simulink model "aircraft_control_model_v2"  (R2020b)
settings: Solver=ode1be  StartTime=0.0  StopTime=t  RelTol=1e-3
values from neighbouring files (symbols this model uses):
  A_ce_CG_14 = A_ce_CG_14(2:3,2:3)    [aircraft_control_model_initialisation_v2.m]
  A_ce_CG_24 = A_ce_CG_24(2:3,2:3)    [aircraft_control_model_initialisation_v2.m]
  A_ce_CG_34 = A_ce_CG_34(2:3,2:3)    [aircraft_control_model_initialisation_v2.m]
  A_sc_CG_10 = A_sc_CG_10(2:3,2:3)    [aircraft_control_model_initialisation_v2.m]
  A_sc_CG_22 = A_sc_CG_22(2:3,2:3)    [aircraft_control_model_initialisation_v2.m]
  A_sc_CG_29 = A_sc_CG_29(2:3,2:3)    [aircraft_control_model_initialisation_v2.m]
  A_sc_CG_36 = A_sc_CG_36(2:3,2:3)    [aircraft_control_model_initialisation_v2.m]
  A_sc_CG_55 = A_sc_CG_55(2:3,2:3)    [aircraft_control_model_initialisation_v2.m]
  actuator_rate = 115*pi/180    (= 2.00712863979)    [aircraft_control_model_initialisation_v2.m]
  ail_sat = 30*pi/180    (= 0.523598775598)    [aircraft_control_model_initialisation_v2.m]
  alpha0 = base_scout_aircraft_constants(16)    [aircraft_control_model_initialisation_v2.m]
  alpha0_ce = base_cessna_aircraft_constants(16)    [aircraft_control_model_initialisation_v2.m]
  alpha0tot_ce_CG_14 = consts_ce_CG_14(17)    [aircraft_control_model_initialisation_v2.m]
  alpha0tot_ce_CG_24 = consts_ce_CG_24(17)    [aircraft_control_model_initialisation_v2.m]
  alpha0tot_ce_CG_34 = consts_ce_CG_34(17)    [aircraft_control_model_initialisation_v2.m]
  alpha0tot_sc_CG_10 = consts_sc_CG_10(17)    [aircraft_control_model_initialisation_v2.m]
  alpha0tot_sc_CG_22 = consts_sc_CG_22(17)    [aircraft_control_model_initialisation_v2.m]
  alpha0tot_sc_CG_29 = consts_sc_CG_29(17)    [aircraft_control_model_initialisation_v2.m]
  alpha0tot_sc_CG_36 = consts_sc_CG_36(17)    [aircraft_control_model_initialisation_v2.m]
  alpha0tot_sc_CG_55 = consts_sc_CG_55(17)    [aircraft_control_model_initialisation_v2.m]
  alpha_ts = base_scout_aircraft_constants(19)    [aircraft_control_model_initialisation_v2.m]
  alpha_ts_ce = base_cessna_aircraft_constants(19)    [aircraft_control_model_initialisation_v2.m]
  alpha_ws = base_scout_aircraft_constants(18)    [aircraft_control_model_initialisation_v2.m]
  alpha_ws_ce = base_cessna_aircraft_constants(18)    [aircraft_control_model_initialisation_v2.m]
  AR_w = base_scout_aircraft_constants(8)    [aircraft_control_model_initialisation_v2.m]
  AR_w_ce = base_cessna_aircraft_constants(8)    [aircraft_control_model_initialisation_v2.m]
  b1 = base_scout_aircraft_constants(23)    [aircraft_control_model_initialisation_v2.m]
  b1_ce = base_cessna_aircraft_constants(23)    [aircraft_control_model_initialisation_v2.m]
  b2 = base_scout_aircraft_constants(24)    [aircraft_control_model_initialisation_v2.m]
  b2_ce = base_cessna_aircraft_constants(24)    [aircraft_control_model_initialisation_v2.m]
  b3 = base_scout_aircraft_constants(25)    [aircraft_control_model_initialisation_v2.m]
  b3_ce = base_cessna_aircraft_constants(25)    [aircraft_control_model_initialisation_v2.m]
  B_ce_CG_14 = B_ce_CG_14(2:3,1:1)    [aircraft_control_model_initialisation_v2.m]
  B_ce_CG_24 = B_ce_CG_24(2:3,1:1)    [aircraft_control_model_initialisation_v2.m]
  B_ce_CG_34 = B_ce_CG_34(2:3,1:1)    [aircraft_control_model_initialisation_v2.m]
  B_sc = B_sc(:,1)    [aircraft_control_model_initialisation_v2.m]
  B_sc_CG_10 = B_sc_CG_10(2:3,1:1)    [aircraft_control_model_initialisation_v2.m]
  B_sc_CG_22 = B_sc_CG_22(2:3,1:1)    [aircraft_control_model_initialisation_v2.m]
  B_sc_CG_29 = B_sc_CG_29(2:3,1:1)    [aircraft_control_model_initialisation_v2.m]
  B_sc_CG_36 = B_sc_CG_36(2:3,1:1)    [aircraft_control_model_initialisation_v2.m]
  B_sc_CG_55 = B_sc_CG_55(2:3,1:1)    [aircraft_control_model_initialisation_v2.m]
  beta_ce_CG_14 = consts_ce_CG_14(21)    [aircraft_control_model_initialisation_v2.m]
  beta_ce_CG_24 = consts_ce_CG_24(21)    [aircraft_control_model_initialisation_v2.m]
  beta_ce_CG_34 = consts_ce_CG_34(21)    [aircraft_control_model_initialisation_v2.m]
  beta_sc_CG_10 = consts_sc_CG_10(21)    [aircraft_control_model_initialisation_v2.m]
  beta_sc_CG_22 = consts_sc_CG_22(21)    [aircraft_control_model_initialisation_v2.m]
  beta_sc_CG_29 = consts_sc_CG_29(21)    [aircraft_control_model_initialisation_v2.m]
  beta_sc_CG_36 = consts_sc_CG_36(21)    [aircraft_control_model_initialisation_v2.m]
  beta_sc_CG_55 = consts_sc_CG_55(21)    [aircraft_control_model_initialisation_v2.m]
  c_e = base_scout_aircraft_constants(10)    [aircraft_control_model_initialisation_v2.m]
  c_e_ce = base_cessna_aircraft_constants(10)    [aircraft_control_model_initialisation_v2.m]
  Cm0 = base_scout_aircraft_constants(11)    [aircraft_control_model_initialisation_v2.m]
  control_surface_feedback = 10    [aircraft_control_model_initialisation_v2.m]
  dCL_w_dalpha = base_scout_aircraft_constants(14)    [aircraft_control_model_initialisation_v2.m]
  dCL_w_dalpha_ce = base_cessna_aircraft_constants(14)    [aircraft_control_model_initialisation_v2.m]
  dCLtot_dalpha = base_scout_aircraft_constants(15)    [aircraft_control_model_initialisation_v2.m]
  dCLtot_dalpha_ce = base_cessna_aircraft_constants(15)    [aircraft_control_model_initialisation_v2.m]
  dt = 1/100    (= 0.01)    [aircraft_control_model_initialisation_v2.m]
  elev_amplitude = 15*pi/180    (= 0.261799387799)    [aircraft_control_model_initialisation_v2.m]
  elev_cutoff = 35*pi/180    (= 0.610865238198)    [aircraft_control_model_initialisation_v2.m]
  elev_period = 1    [aircraft_control_model_initialisation_v2.m]
  elev_period_start = 5    [aircraft_control_model_initialisation_v2.m]
  elev_sat = 28*pi/180    (= 0.488692190558)    [aircraft_control_model_initialisation_v2.m]
  eta_ce_CG_14 = consts_ce_CG_14(22)    [aircraft_control_model_initialisation_v2.m]
  eta_ce_CG_24 = consts_ce_CG_24(22)    [aircraft_control_model_initialisation_v2.m]
  eta_ce_CG_34 = consts_ce_CG_34(22)    [aircraft_control_model_initialisation_v2.m]
  eta_sc_CG_10 = consts_sc_CG_10(22)    [aircraft_control_model_initialisation_v2.m]
  eta_sc_CG_22 = consts_sc_CG_22(22)    [aircraft_control_model_initialisation_v2.m]
  eta_sc_CG_29 = consts_sc_CG_29(22)    [aircraft_control_model_initialisation_v2.m]
  eta_sc_CG_36 = consts_sc_CG_36(22)    [aircraft_control_model_initialisation_v2.m]
  eta_sc_CG_55 = consts_sc_CG_55(22)    [aircraft_control_model_initialisation_v2.m]
  g = base_scout_aircraft_constants(3)    [aircraft_control_model_initialisation_v2.m]
  G = base_scout_aircraft_constants(26)    [aircraft_control_model_initialisation_v2.m]
  g_ce = base_cessna_aircraft_constants(3)    [aircraft_control_model_initialisation_v2.m]
  G_ce = base_cessna_aircraft_constants(26)    [aircraft_control_model_initialisation_v2.m]
  h0 = base_scout_aircraft_constants(13)    [aircraft_control_model_initialisation_v2.m]
  h_cg = base_scout_aircraft_constants(12)    [aircraft_control_model_initialisation_v2.m]
  K = base_scout_aircraft_constants(7)    [aircraft_control_model_initialisation_v2.m]
  l_m = base_scout_aircraft_constants(27)    [aircraft_control_model_initialisation_v2.m]
  l_m_ce = base_cessna_aircraft_constants(27)    [aircraft_control_model_initialisation_v2.m]
  m = base_scout_aircraft_constants(2)    [aircraft_control_model_initialisation_v2.m]
  m_ce = base_cessna_aircraft_constants(2)    [aircraft_control_model_initialisation_v2.m]
  modM = base_scout_aircraft_constants(30)    [aircraft_control_model_initialisation_v2.m]
  modM_ce = base_cessna_aircraft_constants(30)    [aircraft_control_model_initialisation_v2.m]
  n = base_scout_aircraft_constants(1)    [aircraft_control_model_initialisation_v2.m]    (also in xplane_data_decoder.m = data_input(6,2))
  ppgain_actuator_D = 1.076123507883140e+02    (= 107.612350788)    [aircraft_control_model_initialisation_v2.m]
  ppgain_actuator_P = 20.729870007825970    (= 20.7298700078)    [aircraft_control_model_initialisation_v2.m]
  ppgain_D = 0.637114873357555    (= 0.637114873358)    [aircraft_control_model_initialisation_v2.m]
  ppgain_P = -86.717674561182620    (= -86.7176745612)    [aircraft_control_model_initialisation_v2.m]
  r = base_scout_aircraft_constants(29)    [aircraft_control_model_initialisation_v2.m]
  r_ce = base_cessna_aircraft_constants(29)    [aircraft_control_model_initialisation_v2.m]
  rho = base_scout_aircraft_constants(4)    [aircraft_control_model_initialisation_v2.m]
  rho_ce = base_cessna_aircraft_constants(4)    [aircraft_control_model_initialisation_v2.m]
  rud_sat = 28*pi/180    (= 0.488692190558)    [aircraft_control_model_initialisation_v2.m]
  s_e = base_scout_aircraft_constants(9)    [aircraft_control_model_initialisation_v2.m]
  s_e_ce = base_cessna_aircraft_constants(9)    [aircraft_control_model_initialisation_v2.m]
  s_tp = base_scout_aircraft_constants(6)    [aircraft_control_model_initialisation_v2.m]
  s_w = base_scout_aircraft_constants(5)    [aircraft_control_model_initialisation_v2.m]
  s_w_ce = base_cessna_aircraft_constants(5)    [aircraft_control_model_initialisation_v2.m]
  tr = base_scout_aircraft_constants(28)    [aircraft_control_model_initialisation_v2.m]
  tr_ce = base_cessna_aircraft_constants(28)    [aircraft_control_model_initialisation_v2.m]
undefined symbols (not defined in the file or in its folder): A_sc
libraries: simulink x6, pid_lib x4, etargetslib x2, dspnetwork x2, aerolibanimutils x1, sldrtlib x1, cstblocks x1
(part 2 of 3)

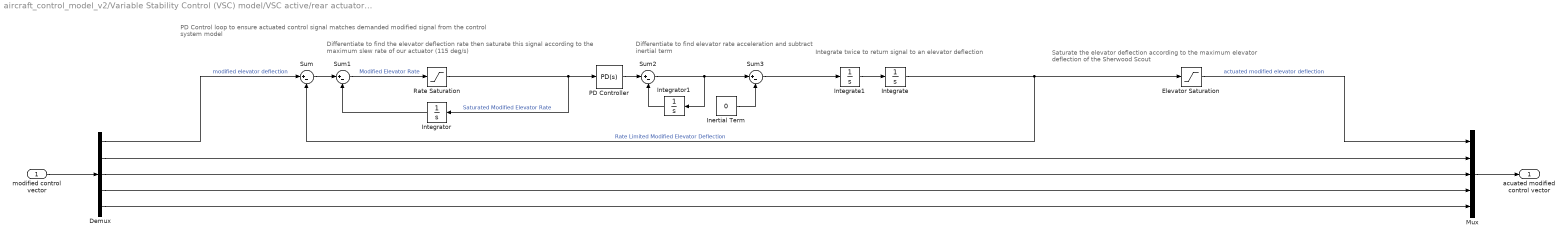
== system aircraft_control_model_v2/Variable Stability Control (VSC) model/VSC active/rear actuator model ==
  note: Differentiate to find the elevator deflection rate then saturate this signal according to the maximum slew rate of our actuator (115 deg/s)
  note: Integrate twice to return signal to an elevator deflection
  note: Saturate the elevator deflection according to the maximum elevator deflection of the Sherwood Scout
  note: PD Control loop to ensure actuated control signal matches demanded modified signal from the control system model
  note: Differentiate to find elevator rate acceleration and subtract inertial term
  modified control vector : Inport
  Demux : Demux  Outputs=5
  Elevator Saturation : Saturate  UpperLimit=elev_sat  LowerLimit=-elev_sat
  Inertial Term : Constant  Value=0
  Integrate : Integrator
  Integrate1 : Integrator
  Integrator : Integrator
  Integrator1 : Integrator
  Mux : Mux  Inputs=5
  PD Controller : pid_lib/PID Controller  Controller=PD  Form=Parallel  TimeDomain=Continuous-time  UseExternalTs=off  SampleTime=-1  IntegratorMethod=Forward Euler  FilterMethod=Forward Euler  ControllerParametersSource=internal  P=ppgain_actuator_P  I=0  D=ppgain_actuator_D  UseFilter=on  N=100  TunerSelectOption=Transfer Function Based (PID Tuner App)  InitialConditionSource=internal  InitialConditionForIntegrator=0  InitialConditionForFilter=0  DifferentiatorICPrevScaledInput=0  ExternalReset=none  TrackingMode=off  Kt=1  LimitOutput=off  SatLimitsSource=internal  UpperSaturationLimit=inf  LowerSaturationLimit=-inf  LinearizeAsGain=on  AntiWindupMode=none  Kb=1  POutMin=[]  POutMax=[]  IOutMin=[]  IOutMax=[]  DOutMin=[]  DOutMax=[]  NOutMin=[]  NOutMax=[]  SumOutMin=[]  SumOutMax=[]  SaturationOutMin=[]  SaturationOutMax=[]  PParamMin=[]  PParamMax=[]  IParamMin=[]  IParamMax=[]  DParamMin=[]  DParamMax=[]  NParamMin=[]  NParamMax=[]  KbParamMin=[]  KbParamMax=[]  KtParamMin=[]  KtParamMax=[]  KbOutMin=[]  KbOutMax=[]  KtOutMin=[]  KtOutMax=[]  IntegratorOutMin=[]  IntegratorOutMax=[]  FilterOutMin=[]  FilterOutMax=[]  SumI1OutMin=[]  SumI1OutMax=[]  SumI2OutMin=[]  SumI2OutMax=[]  SumI3OutMin=[]  SumI3OutMax=[]  SumI4OutMin=[]  SumI4OutMax=[]  SumDOutMin=[]  SumDOutMax=[]  DifferentiatorOutMin=[]  DifferentiatorOutMax=[]  FilterDiffOutCoefMin=[]  FilterDiffOutCoefMax=[]  ReciprocalOutMin=[]  ReciprocalOutMax=[]  SumDenOutMin=[]  SumDenOutMax=[]  SumNumOutMin=[]  SumNumOutMax=[]  DivideOutMin=[]  DivideOutMax=[]  UdiffTsProdOutMin=[]  UdiffTsProdOutMax=[]  NTsProdOutMin=[]  NTsProdOutMax=[]  UintegralTsProdOutMin=[]  UintegralTsProdOutMax=[]  UngainTsProdOutMin=[]  UngainTsProdOutMax=[]  IntegratorContinuousStateAttributes=''  IntegratorStateMustResolveToSignalObject=off  IntegratorRTWStateStorageClass=Auto  FilterContinuousStateAttributes=''  FilterStateMustResolveToSignalObject=off  FilterRTWStateStorageClass=Auto  ParallelPVariant=InternalParameters  IdealPVariant=Disabled  IVariant=Disabled  DVariant=InternalParameters  IntegratorVariant=Disabled  SatVariant=Disabled  AWVariant=Disabled  PCopyVariant=Disabled  TRVariant=Disabled  FdbkBlocksVariant=Forward  IdealPFdbkVariant=Disabled  SatFdbkVariant=Disabled  DerivativeFilterVariant=ContFilter  NVariant=InternalParameters  NCopyVariant=Disabled  FilterICVariant=InternalICsFilter  IntegratorICVariant=Disabled  ExternalResetVariant=Disabled  TRSumVariant=Passthrough  SumFdbkVariant=Disabled  SumVariant=Sum_PD  TsampFilterVariant=InternalTs  TsampNgainVariant=Passthrough  TsampIntegralVariant=Disabled_SignalSpec  ExternalSaturationOutDataTypeStr=Inherit: Same as second input
  Rate Saturation : Saturate  UpperLimit=actuator_rate  LowerLimit=-actuator_rate
  Sum{,1..3} (4 alike) : Sum  Inputs=|+-
  acuated modified control vector : Outport
  wires:
  Demux/1 -> Sum/1  "modified elevator deflection"
  Elevator Saturation/1 -> Mux/1  "actuated modified elevator deflection"
  Rate Saturation/1 -> Integrator/1, PD Controller/1  "Saturated Modified Elevator Rate"
  Integrate/1 -> Sum/2, Elevator Saturation/1  "Rate Limited Modified Elevator Deflection"
  Sum/1 -> Sum1/1
  Sum1/1 -> Rate Saturation/1  "Modified Elevator Rate"
  Integrator/1 -> Sum1/2
  Integrator1/1 -> Sum2/2
  PD Controller/1 -> Sum2/1
  Sum2/1 -> Sum3/1, Integrator1/1
  Inertial Term/1 -> Sum3/2
  Sum3/1 -> Integrate1/1
  Integrate1/1 -> Integrate/1
  modified control vector/1 -> Demux/1
  Demux/2 -> Mux/2
  Demux/3 -> Mux/3
  Demux/4 -> Mux/4
  Demux/5 -> Mux/5
  Mux/1 -> acuated modified control vector/1

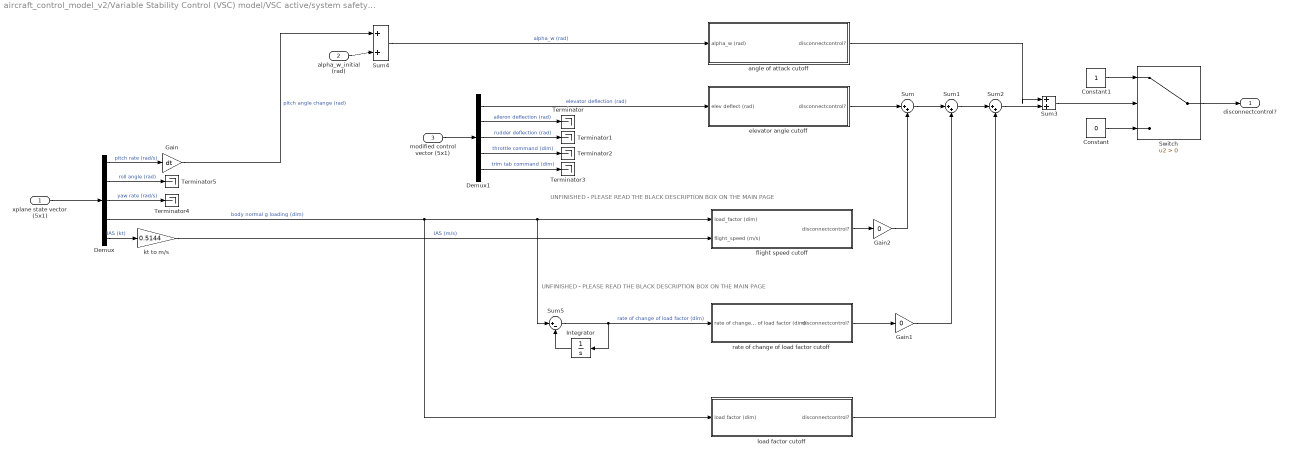
== system aircraft_control_model_v2/Variable Stability Control (VSC) model/VSC active/system safety cutoffs ==
  note: UNFINISHED - PLEASE READ THE BLACK DESCRIPTION BOX ON THE MAIN PAGE
  note: UNFINISHED - PLEASE READ THE BLACK DESCRIPTION BOX ON THE MAIN PAGE
  xplane state vector (5x1) : Inport
  alpha_w_initial (rad) : Inport  Port=2
  modified control vector (5x1) : Inport  Port=3
  Constant : Constant  Value=0
  Constant1 : Constant
  Demux : Demux  Outputs=5
  Demux1 : Demux  Outputs=5
  Gain : Gain  Gain=dt
  Gain1 : Gain  Gain=0
  Gain2 : Gain  Gain=0
  Integrator : Integrator
  Sum{,1..4} (5 alike) : Sum  Inputs=|++
  Sum5 : Sum  Inputs=|+-
  Switch : Switch  Criteria=u2 > Threshold
  Terminator{,1..5} (6 alike) : Terminator
  angle of attack cutoff : Subsystem
  elevator angle cutoff : Subsystem
  flight speed cutoff : Subsystem
  kt to m/s : Gain  Gain=0.5144
  load factor cutoff : Subsystem
  rate of change of load factor cutoff : Subsystem
  disconnectcontrol? : Outport
  wires:
  elevator angle cutoff/1(disconnectcontrol?) -> Sum/1
  Constant/1 -> Switch/3
  Constant1/1 -> Switch/1
  Switch/1 -> disconnectcontrol?/1
  Sum/1 -> Sum1/1
  Sum1/1 -> Sum2/1
  Sum2/1 -> Sum3/2
  rate of change of load factor cutoff/1(disconnectcontrol?) -> Gain1/1
  load factor cutoff/1(disconnectcontrol?) -> Sum2/2
  angle of attack cutoff/1(disconnectcontrol?) -> Sum3/1
  Sum4/1 -> angle of attack cutoff/1(alpha_w (rad))  "alpha_w (rad)"
  xplane state vector (5x1)/1 -> Demux/1
  Demux/1 -> Gain/1  "pitch rate (rad/s)"
  Demux/4 -> load factor cutoff/1(load factor (dim)), Sum5/1, flight speed cutoff/1(load_factor (dim))  "body normal g loading (dim)"
  Demux/2 -> Terminator5/1  "roll angle (rad)"
  Demux/3 -> Terminator4/1  "yaw rate (rad/s)"
  Demux/5 -> kt to m/s/1  "IAS (kt)"
  kt to m/s/1 -> flight speed cutoff/2(flight_speed (m/s))  "IAS (m/s)"
  modified control vector (5x1)/1 -> Demux1/1
  Demux1/1 -> elevator angle cutoff/1(elev deflect (rad))  "elevator deflection (rad)"
  Demux1/2 -> Terminator/1  "aileron deflection (rad)"
  Demux1/3 -> Terminator1/1  "rudder deflection (rad)"
  Demux1/4 -> Terminator2/1  "throttle command (dim)"
  Demux1/5 -> Terminator3/1  "trim tab command (dim)"
  alpha_w_initial (rad)/1 -> Sum4/2
  Gain/1 -> Sum4/1  "pitch angle change (rad)"
  Integrator/1 -> Sum5/2
  Sum5/1 -> Integrator/1, rate of change of load factor cutoff/1(rate of change of load factor (dim))  "rate of change of load factor (dim)"
  flight speed cutoff/1(disconnectcontrol?) -> Gain2/1
  Sum3/1 -> Switch/2
  Gain1/1 -> Sum1/2
  Gain2/1 -> Sum/2

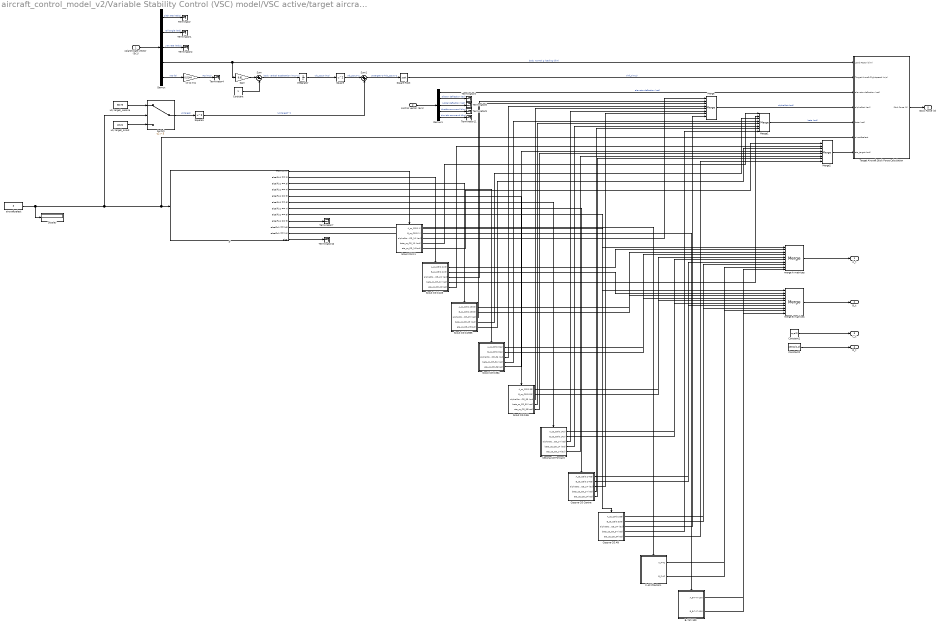
== system aircraft_control_model_v2/Variable Stability Control (VSC) model/VSC active/target aircraft state space selection ==
  xplane state vector (5x1) : Inport
  control vector (5x1) : Inport  Port=2
  B-747-100 : Subsystem  TreatAsAtomicUnit=on
  Cessna CG Aft : Subsystem  TreatAsAtomicUnit=on
  Cessna CG Centre : Subsystem  TreatAsAtomicUnit=on
  Cessna CG Forward : Subsystem  TreatAsAtomicUnit=on
  Constant : Constant
  Constant1 : Constant  Value=eye(2)
  Constant2 : Constant  Value=zeros(1,2)
  Demux : Demux  Outputs=5
  Demux1 : Demux  Outputs=5
  Display : Display
  F-4C Phantom : Subsystem  TreatAsAtomicUnit=on
  Gain : Gain  Gain=9.81
  If : If  IfExpression=u1 == 1  ElseIfExpressions=u1 == 2, u1 == 3, u1 == 4, u1 == 5, u1 == 6, u1 == 7, u1 == 8, u1 == 9, u1 == 10, u1 == 11
  Integrator : Integrator
  Merge : Merge  Inputs=8
  Merge1 : Merge  Inputs=8
  Merge2 : Merge  Inputs=8
  Scout CG 0.1 : Subsystem  TreatAsAtomicUnit=on
  Scout CG 0.223 : Subsystem  TreatAsAtomicUnit=on
  Scout CG 0.2935 : Subsystem  TreatAsAtomicUnit=on
  Scout CG 0.364 : Subsystem  TreatAsAtomicUnit=on
  Scout CG 0.55 : Subsystem  TreatAsAtomicUnit=on
  Square : Math  Operator=square  SaturateOnIntegerOverflow=on
  Square Root : Sqrt  SaturateOnIntegerOverflow=on
  Square1 : Math  Operator=square  SaturateOnIntegerOverflow=on
  Sum : Sum  Inputs=|+-
  Sum1 : Sum  Inputs=|++
  Switch : Switch  Criteria=u2 > Threshold  Threshold=5
  Target Aircraft Stick Force Calculation : Subsystem
  Terminator{,1..4,7..11} (10 alike) : Terminator
  aircraftselect : Constant  Value=3
  kt to m/s : Gain  Gain=0.5144
  merge A matrices : Merge  Inputs=10
  merge B matrices : Merge  Inputs=10
  "u0, target_cessna" : Constant  Value=66.75
  "u0, target_scout" : Constant  Value=43.21
  A_t : Outport
  B_t : Outport  Port=2
  C_t : Outport  Port=3
  D_t : Outport  Port=4
  Stick Force (N) : Outport  Port=5
  wires:
  If/1 -> Scout CG 0.1/Action
  If/2 -> Scout CG 0.223/Action
  If/3 -> Scout CG 0.2935/Action
  If/4 -> Scout CG 0.364/Action
  If/5 -> Scout CG 0.55/Action
  If/6 -> Cessna CG Forward/Action
  If/7 -> Cessna CG Centre/Action
  If/8 -> Cessna CG Aft/Action
  If/9 -> Terminator7/1
  If/10 -> F-4C Phantom/Action
  If/11 -> B-747-100/Action
  If/12 -> Terminator10/1
  Scout CG 0.1/1(A_sc_CG(0.1)) -> merge A matrices/1
  Scout CG 0.223/1(A_sc_CG(0.223)) -> merge A matrices/2
  merge A matrices/1 -> A_t/1
  merge B matrices/1 -> B_t/1
  Scout CG 0.1/2(B_sc_CG(0.1)) -> merge B matrices/1
  Scout CG 0.223/2(B_sc_CG(0.223)) -> merge B matrices/2
  Constant1/1 -> C_t/1
  Constant2/1 -> D_t/1
  aircraftselect/1 -> Display/1, If/1, Target Aircraft Stick Force Calculation/6(aircraftselect), Switch/2
  Scout CG 0.2935/1(A_sc_CG(0.2935)) -> merge A matrices/3
  Scout CG 0.2935/2(B_sc_CG(0.2935)) -> merge B matrices/3
  Scout CG 0.364/1(A_sc_CG(0.364)) -> merge A matrices/4
  Scout CG 0.364/2(B_sc_CG(0.364)) -> merge B matrices/4
  Scout CG 0.55/1(A_sc_CG(0.55)) -> merge A matrices/5
  Scout CG 0.55/2(B_sc_CG(0.55)) -> merge B matrices/5
  xplane state vector (5x1)/1 -> Demux/1
  Demux/5 -> kt to m/s/1  "IAS (kt)"
  Demux/1 -> Terminator/1  "pitch rate (rad/s)"
  Demux/2 -> Terminator1/1  "roll angle (rad)"
  Demux/3 -> Terminator2/1  "yaw rate (rad/s)"
  Demux/4 -> Target Aircraft Stick Force Calculation/1(Load Factor (dim)), Gain/1  "body normal g loading (dim)"
  kt to m/s/1 -> Terminator4/1  "IAS (m/s)"
  control vector (5x1)/1 -> Demux1/1
  Demux1/1 -> Target Aircraft Stick Force Calculation/3(elevator deflection (rad))  "elevator deflection (rad)"
  Demux1/2 -> Terminator3/1  "aileron deflection (rad)"
  Demux1/3 -> Terminator8/1  "rudder deflection (rad)"
  Demux1/4 -> Terminator9/1  "throttle command (dim)"
  Demux1/5 -> Terminator11/1  "trim tab command (dim)"
  Merge/1 -> Target Aircraft Stick Force Calculation/4(alpha0tot (rad))  "alpha0tot (rad)"
  Merge1/1 -> Target Aircraft Stick Force Calculation/5(beta (rad))  "beta (rad)"
  Scout CG 0.223/3(alpha0tot_sc_CG_22 (rad)) -> Merge/2
  Scout CG 0.1/3(alpha0tot_sc_CG_10 (rad)) -> Merge/1
  Scout CG 0.2935/3(alpha0tot_sc_CG_29 (rad)) -> Merge/3
  Scout CG 0.364/3(alpha0tot_sc_CG_36 (rad)) -> Merge/4
  Scout CG 0.55/3(alpha0tot_sc_CG_55 (rad)) -> Merge/5
  Scout CG 0.1/4(beta_sc_CG_10 (rad)) -> Merge1/1
  Scout CG 0.223/4(beta_sc_CG_22 (rad)) -> Merge1/2
  Scout CG 0.2935/4(beta_sc_CG_29 (rad)) -> Merge1/3
  Scout CG 0.364/4(beta_sc_CG_36 (rad)) -> Merge1/4
  Scout CG 0.55/4(beta_sc_CG_55 (rad)) -> Merge1/5
  Target Aircraft Stick Force Calculation/1(Stick Force (N)) -> Stick Force (N)/1
  Cessna CG Forward/1(A_ce_CG(0.143)) -> merge A matrices/6
  Cessna CG Centre/1(A_ce_CG(0.2405)) -> merge A matrices/7
  Cessna CG Aft/1(A_ce_CG(0.338)) -> merge A matrices/8
  F-4C Phantom/1(A_F-4C) -> merge A matrices/9
  B-747-100/1(A_B-747-100) -> merge A matrices/10
  Cessna CG Forward/2(B_ce_CG(0.143)) -> merge B matrices/6
  Cessna CG Centre/2(B_ce_CG(0.2405)) -> merge B matrices/7
  Cessna CG Aft/2(B_ce_CG(0.338)) -> merge B matrices/8
  F-4C Phantom/2(B_F-4C) -> merge B matrices/9
  B-747-100/2(B_B-747-100) -> merge B matrices/10
  Cessna CG Forward/3(alpha0tot_ce_CG_14 (rad)) -> Merge/6
  Cessna CG Centre/3(alpha0tot_ce_CG_24 (rad)) -> Merge/7
  Cessna CG Aft/3(alpha0tot_ce_CG_34 (rad)) -> Merge/8
  Cessna CG Forward/4(beta_ce_CG_14 (rad)) -> Merge1/6
  Cessna CG Centre/4(beta_ce_CG_24 (rad)) -> Merge1/7
  Cessna CG Aft/4(beta_ce_CG_34 (rad)) -> Merge1/8
  Merge2/1 -> Target Aircraft Stick Force Calculation/7(eta_target (rad))
  Scout CG 0.1/5(eta_sc_CG_10(rad)) -> Merge2/1
  Scout CG 0.223/5(eta_sc_CG_22(rad)) -> Merge2/2
  Scout CG 0.2935/5(eta_sc_CG_29(rad)) -> Merge2/3
  Scout CG 0.364/5(eta_sc_CG_36(rad)) -> Merge2/4
  Scout CG 0.55/5(eta_sc_CG_55(rad)) -> Merge2/5
  Cessna CG Forward/5(eta_ce_CG_14(rad)) -> Merge2/6
  Cessna CG Centre/5(eta_ce_CG_24(rad)) -> Merge2/7
  Cessna CG Aft/5(eta_ce_CG_34(rad)) -> Merge2/8
  "u0, target_cessna"/1 -> Switch/1
  "u0, target_scout"/1 -> Switch/3
  Switch/1 -> Square1/1  "u0,target"
  Gain/1 -> Sum/1
  Constant/1 -> Sum/2
  Sum/1 -> Integrator/1  "body vertical acceleration (m/s^2)"
  Integrator/1 -> Square/1  "wb_scout (m/s)"
  Square/1 -> Sum1/1  "wb_scout^2"
  Square1/1 -> Sum1/2  "(u0,target)^2"
  Sum1/1 -> Square Root/1  "u0,target^2+wb_scout^2"
  Square Root/1 -> Target Aircraft Stick Force Calculation/2(Target Aircraft Flightspeed (m/s))  "Vinf_t (m/s)"

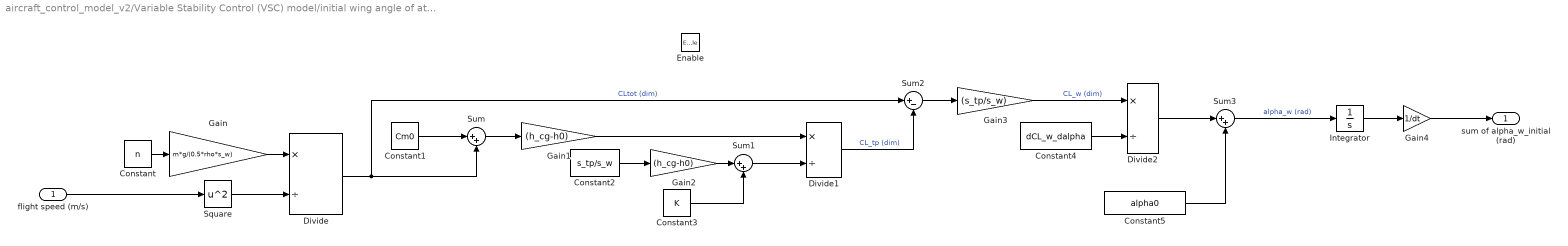
== system aircraft_control_model_v2/Variable Stability Control (VSC) model/initial wing angle of attack (rad) estimation/Enabled Subsystem ==
  flight speed (m/s) : Inport
  Enable : EnablePort
  Constant : Constant  Value=n
  Constant1 : Constant  Value=Cm0
  Constant2 : Constant  Value=s_tp/s_w
  Constant3 : Constant  Value=K
  Constant4 : Constant  Value=dCL_w_dalpha
  Constant5 : Constant  Value=alpha0
  Divide : Product  Inputs=*/
  Divide1 : Product  Inputs=*/
  Divide2 : Product  Inputs=*/
  Gain : Gain  Gain=m*g/(0.5*rho*s_w)
  Gain1 : Gain  Gain=(h_cg-h0)
  Gain2 : Gain  Gain=(h_cg-h0)
  Gain3 : Gain  Gain=(s_tp/s_w)
  Gain4 : Gain  Gain=1/dt
  Integrator : Integrator
  Square : Math  Operator=square  SaturateOnIntegerOverflow=on
  Sum : Sum  Inputs=|++
  Sum1 : Sum  Inputs=|++
  Sum2 : Sum  Inputs=|+-
  Sum3 : Sum  Inputs=|++
  sum of alpha_w_initial (rad) : Outport
  wires:
  Gain1/1 -> Divide1/1
  Gain/1 -> Divide/1
  Gain2/1 -> Sum1/1
  Divide/1 -> Sum2/1, Sum/2  "CLtot (dim)"
  Constant/1 -> Gain/1
  Sum/1 -> Gain1/1
  Constant4/1 -> Divide2/2
  Divide2/1 -> Sum3/1
  Constant3/1 -> Sum1/2
  Sum1/1 -> Divide1/2
  Sum2/1 -> Gain3/1
  Constant1/1 -> Sum/1
  Square/1 -> Divide/2
  Constant2/1 -> Gain2/1
  Gain3/1 -> Divide2/1  "CL_w (dim)"
  Constant5/1 -> Sum3/2
  Sum3/1 -> Integrator/1  "alpha_w (rad)"
  flight speed (m/s)/1 -> Square/1
  Divide1/1 -> Sum2/2  "CL_tp (dim)"
  Integrator/1 -> Gain4/1
  Gain4/1 -> sum of alpha_w_initial (rad)/1

== system aircraft_control_model_v2/Control Inputs/pilot joystick input/control surface commands to control surface deflections/aileron command to aileron deflection ==
  aileron command (dim) : Inport
  Gain2 : Gain  Gain=control_surface_feedback
  Gain3 : Gain  Gain=control_surface_feedback*(ail_sat)
  Integrator4 : Integrator
  Sum1 : Sum  Inputs=|+-
  aileron deflection (rad) : Outport
  wires:
  Gain2/1 -> Sum1/2
  Sum1/1 -> Integrator4/1
  Gain3/1 -> aileron deflection (rad)/1  "aileron deflection (rad)"
  Integrator4/1 -> Gain3/1, Gain2/1
  aileron command (dim)/1 -> Sum1/1

== system aircraft_control_model_v2/Control Inputs/pilot joystick input/control surface commands to control surface deflections/elevator command to elevator deflection ==
  elevator command (dim) : Inport
  Gain : Gain  Gain=control_surface_feedback
  Gain1 : Gain  Gain=control_surface_feedback*(elev_sat)
  Gain2 : Gain  Gain=-1
  Integrator1 : Integrator
  Sum : Sum  Inputs=|+-
  elevator deflection (rad) : Outport
  wires:
  Integrator1/1 -> Gain/1, Gain1/1
  Gain1/1 -> elevator deflection (rad)/1  "elevator deflection (rad)"
  Sum/1 -> Integrator1/1
  Gain/1 -> Sum/2
  elevator command (dim)/1 -> Gain2/1
  Gain2/1 -> Sum/1

== system aircraft_control_model_v2/Control Inputs/pilot joystick input/control surface commands to control surface deflections/rudder command to rudder deflection ==
  rudder command (dim) : Inport
  Gain4 : Gain  Gain=control_surface_feedback
  Gain5 : Gain  Gain=control_surface_feedback*(rud_sat)
  Integrator3 : Integrator
  Sum2 : Sum  Inputs=|+-
  rudder deflection (rad) : Outport
  wires:
  Integrator3/1 -> Gain5/1, Gain4/1
  Gain5/1 -> rudder deflection (rad)/1  "rudder deflection (rad)"
  Sum2/1 -> Integrator3/1
  Gain4/1 -> Sum2/2
  rudder command (dim)/1 -> Sum2/1

== system aircraft_control_model_v2/Variable Stability Control (VSC) model/VSC active/system safety cutoffs/angle of attack cutoff ==
  alpha_w (rad) : Inport
  +ve wing angle of attack limit (rad) : simulink/Logic and Bit Operations/Compare To Constant  relop=>  const=10*pi/180  OutDataTypeStr=boolean
  -ve wing angle of attack limit (rad) : simulink/Logic and Bit Operations/Compare To Constant  relop=<  const=-7*pi/180  OutDataTypeStr=boolean
  Constant : Constant  Value=0
  Constant1 : Constant
  Logical Operator : Logic  Operator=OR  AllPortsSameDT=off  OutDataTypeStr=boolean
  Logical Operator1 : Logic  Operator=OR  AllPortsSameDT=off  OutDataTypeStr=boolean
  Memory : Memory
  Memory1 : Memory
  Sum : Sum  Inputs=|++
  Switch : Switch  Criteria=u2 > Threshold
  disconnectcontrol? : Outport
  wires:
  Constant/1 -> Switch/3
  Constant1/1 -> Switch/1
  Logical Operator/1 -> Sum/1, Memory/1
  Memory/1 -> Logical Operator/1
  Sum/1 -> Switch/2
  Logical Operator1/1 -> Sum/2, Memory1/1
  +ve wing angle of attack limit (rad)/1 -> Logical Operator/2
  -ve wing angle of attack limit (rad)/1 -> Logical Operator1/2
  alpha_w (rad)/1 -> -ve wing angle of attack limit (rad)/1, +ve wing angle of attack limit (rad)/1
  Memory1/1 -> Logical Operator1/1
  Switch/1 -> disconnectcontrol?/1

== system aircraft_control_model_v2/Variable Stability Control (VSC) model/VSC active/system safety cutoffs/elevator angle cutoff ==
  elev deflect (rad) : Inport
  Abs : Abs
  Compare To Constant : simulink/Logic and Bit Operations/Compare To Constant  relop=>  const=elev_cutoff  OutDataTypeStr=boolean
  Logical Operator : Logic  Operator=OR  AllPortsSameDT=off  OutDataTypeStr=boolean
  Memory : Memory
  disconnectcontrol? : Outport
  wires:
  Memory/1 -> Logical Operator/1
  elev deflect (rad)/1 -> Abs/1
  Abs/1 -> Compare To Constant/1
  Compare To Constant/1 -> Logical Operator/2
  Logical Operator/1 -> disconnectcontrol?/1, Memory/1

== system aircraft_control_model_v2/Variable Stability Control (VSC) model/VSC active/system safety cutoffs/flight speed cutoff ==
  load_factor (dim) : Inport
  flight_speed (m/s) : Inport  Port=2
  Logical Operator1 : Logic  Operator=OR  AllPortsSameDT=off  OutDataTypeStr=boolean
  MATLAB Function : MATLAB Function  TreatAsAtomicUnit=on
  Memory1 : Memory
  Relational Operator : RelationalOperator  Operator=<  OutDataTypeStr=boolean  RndMeth=Simplest
  disconnectcontrol? : Outport
  wires:
  load_factor (dim)/1 -> MATLAB Function/1(n)  "Load Factor (dim)"
  flight_speed (m/s)/1 -> Relational Operator/1  "flight_speed (m/s)"
  Relational Operator/1 -> Logical Operator1/2
  Memory1/1 -> Logical Operator1/1
  Logical Operator1/1 -> disconnectcontrol?/1, Memory1/1
  MATLAB Function/1(Va) -> Relational Operator/2

== system aircraft_control_model_v2/Variable Stability Control (VSC) model/VSC active/system safety cutoffs/load factor cutoff ==
  load factor (dim) : Inport
  Compare To Constant : simulink/Logic and Bit Operations/Compare To Constant  relop=>  const=3.5  OutDataTypeStr=boolean
  Compare To Constant1 : simulink/Logic and Bit Operations/Compare To Constant  relop=<  const=-1.2  OutDataTypeStr=boolean
  Constant : Constant  Value=0
  Constant1 : Constant
  Logical Operator : Logic  Operator=OR  AllPortsSameDT=off  OutDataTypeStr=boolean
  Logical Operator1 : Logic  Operator=OR  AllPortsSameDT=off  OutDataTypeStr=boolean
  Memory : Memory
  Memory1 : Memory
  Sum : Sum  Inputs=|++
  Switch : Switch  Criteria=u2 > Threshold
  disconnectcontrol? : Outport
  wires:
  load factor (dim)/1 -> Compare To Constant1/1, Compare To Constant/1
  Compare To Constant/1 -> Logical Operator/2
  Memory/1 -> Logical Operator/1
  Logical Operator/1 -> Sum/1, Memory/1
  Compare To Constant1/1 -> Logical Operator1/2
  Memory1/1 -> Logical Operator1/1
  Logical Operator1/1 -> Sum/2, Memory1/1
  Sum/1 -> Switch/2
  Constant1/1 -> Switch/1
  Constant/1 -> Switch/3
  Switch/1 -> disconnectcontrol?/1

== system aircraft_control_model_v2/Variable Stability Control (VSC) model/VSC active/system safety cutoffs/rate of change of load factor cutoff ==
  rate of change of load factor (dim) : Inport
  Abs : Abs
  Compare To Constant : simulink/Logic and Bit Operations/Compare To Constant  relop=>  const=7.8  OutDataTypeStr=boolean
  Logical Operator : Logic  Operator=OR  AllPortsSameDT=off  OutDataTypeStr=boolean
  Memory : Memory
  disconnectcontrol? : Outport
  wires:
  Logical Operator/1 -> disconnectcontrol?/1, Memory/1
  Abs/1 -> Compare To Constant/1
  Compare To Constant/1 -> Logical Operator/2
  Memory/1 -> Logical Operator/1
  rate of change of load factor (dim)/1 -> Abs/1

== system aircraft_control_model_v2/Variable Stability Control (VSC) model/VSC active/target aircraft state space selection/B-747-100 ==
  Action Port : ActionPort  ActionPortLabel=elseif( u1 == 11)
  Constant : Constant  Value=|
      | [-0.508647705600000	65.0870077697200
      | -0.00557351174471139	-0.415074491893133]
  Constant1 : Constant  Value=|
      | [-1.97021509716000
      | -0.377425932894150]
  A_B-747-100 : Outport
  B_B-747-100 : Outport  Port=2
  wires:
  Constant/1 -> A_B-747-100/1
  Constant1/1 -> B_B-747-100/1

== system aircraft_control_model_v2/Variable Stability Control (VSC) model/VSC active/target aircraft state space selection/Cessna CG Aft ==
  Action Port : ActionPort  ActionPortLabel=elseif( u1 == 8)
  Constant : Constant  Value=A_ce_CG_34
  Constant1 : Constant  Value=B_ce_CG_34
  Constant2 : Constant  Value=alpha0tot_ce_CG_34
  Constant3 : Constant  Value=beta_ce_CG_34
  Constant4 : Constant  Value=eta_ce_CG_34
  A_ce_CG(0.338) : Outport
  B_ce_CG(0.338) : Outport  Port=2
  alpha0tot_ce_CG_34 (rad) : Outport  Port=3
  beta_ce_CG_34 (rad) : Outport  Port=4
  eta_ce_CG_34(rad) : Outport  Port=5
  wires:
  Constant/1 -> A_ce_CG(0.338)/1
  Constant1/1 -> B_ce_CG(0.338)/1
  Constant2/1 -> alpha0tot_ce_CG_34 (rad)/1
  Constant3/1 -> beta_ce_CG_34 (rad)/1
  Constant4/1 -> eta_ce_CG_34(rad)/1

== system aircraft_control_model_v2/Variable Stability Control (VSC) model/VSC active/target aircraft state space selection/Cessna CG Centre ==
  Action Port : ActionPort  ActionPortLabel=elseif( u1 == 7)
  Constant : Constant  Value=A_ce_CG_24
  Constant1 : Constant  Value=B_ce_CG_24
  Constant2 : Constant  Value=alpha0tot_ce_CG_24
  Constant3 : Constant  Value=beta_ce_CG_24
  Constant4 : Constant  Value=eta_ce_CG_24
  A_ce_CG(0.2405) : Outport
  B_ce_CG(0.2405) : Outport  Port=2
  alpha0tot_ce_CG_24 (rad) : Outport  Port=3
  beta_ce_CG_24 (rad) : Outport  Port=4
  eta_ce_CG_24(rad) : Outport  Port=5
  wires:
  Constant/1 -> A_ce_CG(0.2405)/1
  Constant1/1 -> B_ce_CG(0.2405)/1
  Constant2/1 -> alpha0tot_ce_CG_24 (rad)/1
  Constant3/1 -> beta_ce_CG_24 (rad)/1
  Constant4/1 -> eta_ce_CG_24(rad)/1

== system aircraft_control_model_v2/Variable Stability Control (VSC) model/VSC active/target aircraft state space selection/Cessna CG Forward ==
  Action Port : ActionPort  ActionPortLabel=elseif( u1 == 6)
  Constant : Constant  Value=A_ce_CG_14
  Constant1 : Constant  Value=B_ce_CG_14
  Constant2 : Constant  Value=alpha0tot_ce_CG_14
  Constant3 : Constant  Value=beta_ce_CG_14
  Constant4 : Constant  Value=eta_ce_CG_14
  A_ce_CG(0.143) : Outport
  B_ce_CG(0.143) : Outport  Port=2
  alpha0tot_ce_CG_14 (rad) : Outport  Port=3
  beta_ce_CG_14 (rad) : Outport  Port=4
  eta_ce_CG_14(rad) : Outport  Port=5
  wires:
  Constant/1 -> A_ce_CG(0.143)/1
  Constant1/1 -> B_ce_CG(0.143)/1
  Constant2/1 -> alpha0tot_ce_CG_14 (rad)/1
  Constant3/1 -> beta_ce_CG_14 (rad)/1
  Constant4/1 -> eta_ce_CG_14(rad)/1

== system aircraft_control_model_v2/Variable Stability Control (VSC) model/VSC active/target aircraft state space selection/F-4C Phantom ==
  Action Port : ActionPort  ActionPortLabel=elseif( u1 == 10)
  Constant : Constant  Value=|
      | [-0.295319442940517	177.255749314106
      | -0.0104482212700093	-0.448358567032906]
  Constant1 : Constant  Value=|
      | [-6.29389106785740
      | -4.88848338612147]
  A_F-4C : Outport
  B_F-4C : Outport  Port=2
  wires:
  Constant/1 -> A_F-4C/1
  Constant1/1 -> B_F-4C/1

== system aircraft_control_model_v2/Variable Stability Control (VSC) model/VSC active/target aircraft state space selection/Scout CG 0.1 ==
  Action Port : ActionPort  ActionPortLabel=if(u1 == 1)
  Constant : Constant  Value=A_sc_CG_10
  Constant1 : Constant  Value=B_sc_CG_10
  Constant2 : Constant  Value=alpha0tot_sc_CG_10
  Constant3 : Constant  Value=beta_sc_CG_10
  Constant4 : Constant  Value=eta_sc_CG_10
  A_sc_CG(0.1) : Outport
  B_sc_CG(0.1) : Outport  Port=2
  alpha0tot_sc_CG_10 (rad) : Outport  Port=3
  beta_sc_CG_10 (rad) : Outport  Port=4
  eta_sc_CG_10(rad) : Outport  Port=5
  wires:
  Constant/1 -> A_sc_CG(0.1)/1
  Constant1/1 -> B_sc_CG(0.1)/1
  Constant2/1 -> alpha0tot_sc_CG_10 (rad)/1
  Constant3/1 -> beta_sc_CG_10 (rad)/1
  Constant4/1 -> eta_sc_CG_10(rad)/1

== system aircraft_control_model_v2/Variable Stability Control (VSC) model/VSC active/target aircraft state space selection/Scout CG 0.223 ==
  Action Port : ActionPort  ActionPortLabel=elseif(u1 == 2)
  Constant : Constant  Value=A_sc_CG_22
  Constant1 : Constant  Value=B_sc_CG_22
  Constant2 : Constant  Value=alpha0tot_sc_CG_22
  Constant3 : Constant  Value=beta_sc_CG_22
  Constant4 : Constant  Value=eta_sc_CG_22
  A_sc_CG(0.223) : Outport
  B_sc_CG(0.223) : Outport  Port=2
  alpha0tot_sc_CG_22 (rad) : Outport  Port=3
  beta_sc_CG_22 (rad) : Outport  Port=4
  eta_sc_CG_22(rad) : Outport  Port=5
  wires:
  Constant/1 -> A_sc_CG(0.223)/1
  Constant1/1 -> B_sc_CG(0.223)/1
  Constant2/1 -> alpha0tot_sc_CG_22 (rad)/1
  Constant3/1 -> beta_sc_CG_22 (rad)/1
  Constant4/1 -> eta_sc_CG_22(rad)/1

== system aircraft_control_model_v2/Variable Stability Control (VSC) model/VSC active/target aircraft state space selection/Scout CG 0.2935 ==
  Action Port : ActionPort  ActionPortLabel=elseif( u1 == 3)
  Constant : Constant  Value=A_sc_CG_29
  Constant1 : Constant  Value=B_sc_CG_29
  Constant2 : Constant  Value=alpha0tot_sc_CG_29
  Constant3 : Constant  Value=beta_sc_CG_29
  Constant4 : Constant  Value=eta_sc_CG_29
  A_sc_CG(0.2935) : Outport
  B_sc_CG(0.2935) : Outport  Port=2
  alpha0tot_sc_CG_29 (rad) : Outport  Port=3
  beta_sc_CG_29 (rad) : Outport  Port=4
  eta_sc_CG_29(rad) : Outport  Port=5
  wires:
  Constant/1 -> A_sc_CG(0.2935)/1
  Constant1/1 -> B_sc_CG(0.2935)/1
  Constant2/1 -> alpha0tot_sc_CG_29 (rad)/1
  Constant3/1 -> beta_sc_CG_29 (rad)/1
  Constant4/1 -> eta_sc_CG_29(rad)/1

== system aircraft_control_model_v2/Variable Stability Control (VSC) model/VSC active/target aircraft state space selection/Scout CG 0.364 ==
  Action Port : ActionPort  ActionPortLabel=elseif( u1 == 4)
  Constant : Constant  Value=A_sc_CG_36
  Constant1 : Constant  Value=B_sc_CG_36
  Constant2 : Constant  Value=alpha0tot_sc_CG_36
  Constant3 : Constant  Value=beta_sc_CG_36
  Constant4 : Constant  Value=eta_sc_CG_36
  A_sc_CG(0.364) : Outport
  B_sc_CG(0.364) : Outport  Port=2
  alpha0tot_sc_CG_36 (rad) : Outport  Port=3
  beta_sc_CG_36 (rad) : Outport  Port=4
  eta_sc_CG_36(rad) : Outport  Port=5
  wires:
  Constant/1 -> A_sc_CG(0.364)/1
  Constant1/1 -> B_sc_CG(0.364)/1
  Constant2/1 -> alpha0tot_sc_CG_36 (rad)/1
  Constant3/1 -> beta_sc_CG_36 (rad)/1
  Constant4/1 -> eta_sc_CG_36(rad)/1

== system aircraft_control_model_v2/Variable Stability Control (VSC) model/VSC active/target aircraft state space selection/Scout CG 0.55 ==
  Action Port : ActionPort  ActionPortLabel=elseif( u1 == 5)
  Constant : Constant  Value=A_sc_CG_55
  Constant1 : Constant  Value=B_sc_CG_55
  Constant2 : Constant  Value=alpha0tot_sc_CG_55
  Constant3 : Constant  Value=beta_sc_CG_55
  Constant4 : Constant  Value=eta_sc_CG_55
  A_sc_CG(0.55) : Outport
  B_sc_CG(0.55) : Outport  Port=2
  alpha0tot_sc_CG_55 (rad) : Outport  Port=3
  beta_sc_CG_55 (rad) : Outport  Port=4
  eta_sc_CG_55(rad) : Outport  Port=5
  wires:
  Constant/1 -> A_sc_CG(0.55)/1
  Constant1/1 -> B_sc_CG(0.55)/1
  Constant2/1 -> alpha0tot_sc_CG_55 (rad)/1
  Constant3/1 -> beta_sc_CG_55 (rad)/1
  Constant4/1 -> eta_sc_CG_55(rad)/1

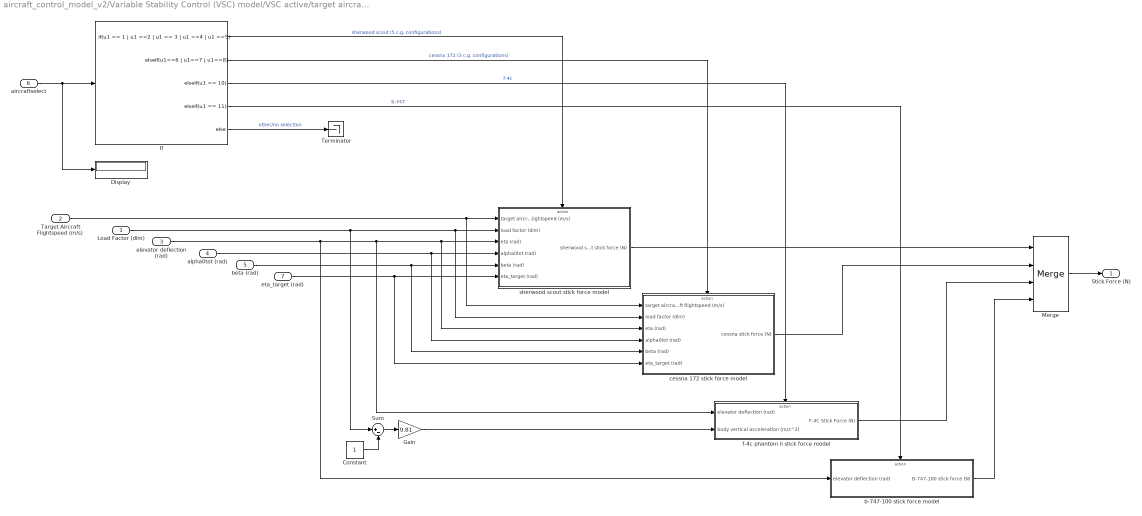
== system aircraft_control_model_v2/Variable Stability Control (VSC) model/VSC active/target aircraft state space selection/Target Aircraft Stick Force Calculation ==
  Load Factor (dim) : Inport
  Target Aircraft Flightspeed (m/s) : Inport  Port=2
  elevator deflection (rad) : Inport  Port=3
  alpha0tot (rad) : Inport  Port=4
  beta (rad) : Inport  Port=5
  aircraftselect : Inport  Port=6
  eta_target (rad) : Inport  Port=7
  Constant : Constant
  Display : Display
  Gain : Gain  Gain=9.81
  If : If  IfExpression=u1 == 1 | u1 ==2 | u1 == 3 | u1 ==4 | u1 ==5  ElseIfExpressions=u1==6 | u1==7 | u1==8,u1 == 10, u1 == 11
  Merge : Merge  Inputs=4
  Sum : Sum  Inputs=|+-
  Terminator : Terminator
  b-747-100 stick force model : Subsystem  TreatAsAtomicUnit=on
  cessna 172 stick force model : Subsystem  TreatAsAtomicUnit=on
  f-4c phantom ii stick force model : Subsystem  TreatAsAtomicUnit=on
  sherwood scout stick force model : Subsystem  TreatAsAtomicUnit=on
  Stick Force (N) : Outport
  wires:
  Merge/1 -> Stick Force (N)/1
  Target Aircraft Flightspeed (m/s)/1 -> cessna 172 stick force model/1(target aircraft flightspeed (m/s)), sherwood scout stick force model/1(target aircraft flightspeed (m/s))
  Load Factor (dim)/1 -> Sum/1, cessna 172 stick force model/2(load factor (dim)), sherwood scout stick force model/2(load factor (dim))
  elevator deflection (rad)/1 -> sherwood scout stick force model/3(eta (rad)), cessna 172 stick force model/3(eta (rad)), f-4c phantom ii stick force model/1(elevator deflection (rad)), b-747-100 stick force model/1(elevator deflection (rad))
  alpha0tot (rad)/1 -> cessna 172 stick force model/4("alpha0tot (rad) "), sherwood scout stick force model/4("alpha0tot (rad) ")
  beta (rad)/1 -> cessna 172 stick force model/5(beta (rad)), sherwood scout stick force model/5(beta (rad))
  aircraftselect/1 -> Display/1, If/1
  If/5 -> Terminator/1  "other/no selection"
  If/1 -> sherwood scout stick force model/Action  "sherwood scout (5 c.g. configurations)"
  If/2 -> cessna 172 stick force model/Action  "cessna 172 (3 c.g. configurations)"
  If/4 -> b-747-100 stick force model/Action  "b-747"
  If/3 -> f-4c phantom ii stick force model/Action  "f-4c"
  cessna 172 stick force model/1(cessna stick force (N)) -> Merge/2
  sherwood scout stick force model/1(sherwood scout stick force (N)) -> Merge/1
  b-747-100 stick force model/1(B-747-100 stick force (N)) -> Merge/4
  eta_target (rad)/1 -> cessna 172 stick force model/6(eta_target (rad)), sherwood scout stick force model/6(eta_target (rad))
  Constant/1 -> Sum/2
  Sum/1 -> Gain/1
  Gain/1 -> f-4c phantom ii stick force model/2(body vertical acceleration (m/s^2))
  f-4c phantom ii stick force model/1(F-4C Stick Force (N)) -> Merge/3

== system aircraft_control_model_v2/Variable Stability Control (VSC) model/VSC active/target aircraft state space selection/Target Aircraft Stick Force Calculation/b-747-100 stick force model ==
  elevator deflection (rad) : Inport
  Action Port : ActionPort  ActionPortLabel=elseif( u1 == 11)
  Subsystem1 : Subsystem
  B-747-100 stick force (N) : Outport
  wires:
  elevator deflection (rad)/1 -> Subsystem1/1(elevator deflection (rad))
  Subsystem1/1(B-747-100 stick force (N)) -> B-747-100 stick force (N)/1  "B-747-100 stick force (N)"

== system aircraft_control_model_v2/Variable Stability Control (VSC) model/VSC active/target aircraft state space selection/Target Aircraft Stick Force Calculation/cessna 172 stick force model ==
  target aircraft flightspeed (m/s) : Inport
  load factor (dim) : Inport  Port=2
  eta (rad) : Inport  Port=3
  "alpha0tot (rad) " : Inport  Port=4
  beta (rad) : Inport  Port=5
  eta_target (rad) : Inport  Port=6
  Action Port : ActionPort  ActionPortLabel=elseif(u1==6 | u1==7 | u1==8)
  Subsystem : Subsystem
  cessna stick force (N) : Outport
  wires:
  Subsystem/1(cessna stick force (N)) -> cessna stick force (N)/1
  target aircraft flightspeed (m/s)/1 -> Subsystem/1(Target Aircraft Flightspeed (m/s))
  load factor (dim)/1 -> Subsystem/2(Load Factor (dim))
  eta (rad)/1 -> Subsystem/3(eta (rad))
  "alpha0tot (rad) "/1 -> Subsystem/4(alpha0tot (rad))
  beta (rad)/1 -> Subsystem/5(beta (rad))
  eta_target (rad)/1 -> Subsystem/6(eta_target (rad))

== system aircraft_control_model_v2/Variable Stability Control (VSC) model/VSC active/target aircraft state space selection/Target Aircraft Stick Force Calculation/f-4c phantom ii stick force model ==
  elevator deflection (rad) : Inport
  body vertical acceleration (m/s^2) : Inport  Port=2
  Action Port : ActionPort  ActionPortLabel=elseif(u1 == 10)
  Gain : Gain  Gain=1/elev_sat
  Gain1 : Gain  Gain=-9.81
  Sum : Sum  Inputs=|+-
  bobweight : Gain  Gain=5.35/32.2
  lb to kg : Gain  Gain=1/2.205
  lb/inch : Gain  Gain=0.7782
  max travel of f-4c stick (inch) : Gain  Gain=4
  F-4C Stick Force (N) : Outport
  wires:
  elevator deflection (rad)/1 -> Gain/1  "elevator deflection (rad)"
  Gain/1 -> max travel of f-4c stick (inch)/1  "elevator command (dim)"
  lb/inch/1 -> Sum/1
  bobweight/1 -> Sum/2
  Sum/1 -> lb to kg/1  "Stick Force (lb)"
  body vertical acceleration (m/s^2)/1 -> bobweight/1
  Gain1/1 -> F-4C Stick Force (N)/1  "Stick Force (N)"
  lb to kg/1 -> Gain1/1  "Stick Force (kg)"
  max travel of f-4c stick (inch)/1 -> lb/inch/1

== system aircraft_control_model_v2/Variable Stability Control (VSC) model/VSC active/target aircraft state space selection/Target Aircraft Stick Force Calculation/sherwood scout stick force model ==
  target aircraft flightspeed (m/s) : Inport
  load factor (dim) : Inport  Port=2
  eta (rad) : Inport  Port=3
  "alpha0tot (rad) " : Inport  Port=4
  beta (rad) : Inport  Port=5
  eta_target (rad) : Inport  Port=6
  Action Port : ActionPort  ActionPortLabel=if(u1 == 1 | u1 ==2 | u1 == 3 | u1 ==4 | u1 ==5)
  Subsystem : Subsystem
  sherwood scout stick force (N) : Outport
  wires:
  Subsystem/1(sherwood scout stick force (N)) -> sherwood scout stick force (N)/1
  target aircraft flightspeed (m/s)/1 -> Subsystem/1(Target Aircraft Flightspeed (m/s))
  load factor (dim)/1 -> Subsystem/2(Load Factor (dim))
  eta (rad)/1 -> Subsystem/3(eta (rad))
  "alpha0tot (rad) "/1 -> Subsystem/4(alpha0tot (rad))
  beta (rad)/1 -> Subsystem/5(beta (rad))
  eta_target (rad)/1 -> Subsystem/6(eta_target (rad))

== system aircraft_control_model_v2/Variable Stability Control (VSC) model/VSC active/target aircraft state space selection/Target Aircraft Stick Force Calculation/b-747-100 stick force model/Subsystem1 ==
  elevator deflection (rad) : Inport
  Gain : Gain  Gain=1/12
  Gain1 : Gain  Gain=9.81
  Gain2 : Gain  Gain=1/elev_sat
  If : If  IfExpression=u1 > 2.5  ElseIfExpressions=u1 < -2.5
  If Action Subsystem : Subsystem  TreatAsAtomicUnit=on
  If Action Subsystem1 : Subsystem  TreatAsAtomicUnit=on
  If Action Subsystem2 : Subsystem  TreatAsAtomicUnit=on
  Merge : Merge  Inputs=3
  Scope1 : Scope
  To Workspace : ToWorkspace  VariableName=b747_stick_force  SaveFormat=Timeseries  SampleTime=-1
  To Workspace1 : ToWorkspace  VariableName=b747_stick_position  SaveFormat=Timeseries  SampleTime=-1
  lb to kg : Gain  Gain=1/2.205
  max b-747-100 column deflection (deg) : Gain  Gain=12
  B-747-100 stick force (N) : Outport
  wires:
  max b-747-100 column deflection (deg)/1 -> Gain/1, If Action Subsystem/1(In1), If Action Subsystem1/1(In1), If Action Subsystem2/1(In1), If/1  "delta_cc (deg)"
  elevator deflection (rad)/1 -> Gain2/1
  Gain2/1 -> max b-747-100 column deflection (deg)/1
  Merge/1 -> lb to kg/1  "F_cc (lb)"
  If Action Subsystem2/1(Out1) -> Merge/3
  If/2 -> If Action Subsystem2/Action
  If/1 -> If Action Subsystem1/Action
  If Action Subsystem1/1(Out1) -> Merge/1
  If/3 -> If Action Subsystem/Action
  lb to kg/1 -> Gain1/1, To Workspace/1, Scope1/1  "F_cc (kg)"
  If Action Subsystem/1(Out1) -> Merge/2
  Gain/1 -> To Workspace1/1
  Gain1/1 -> B-747-100 stick force (N)/1

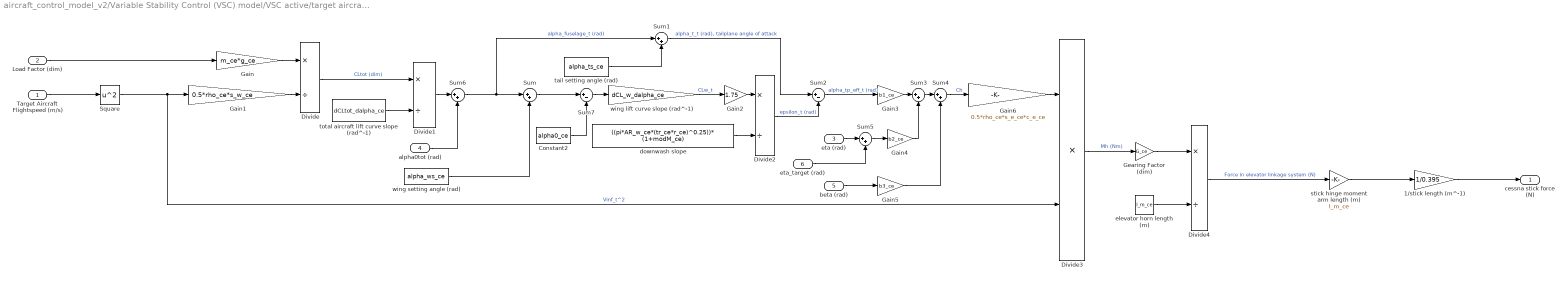
== system aircraft_control_model_v2/Variable Stability Control (VSC) model/VSC active/target aircraft state space selection/Target Aircraft Stick Force Calculation/cessna 172 stick force model/Subsystem ==
  Target Aircraft Flightspeed (m/s) : Inport
  Load Factor (dim) : Inport  Port=2
  eta (rad) : Inport  Port=3
  alpha0tot (rad) : Inport  Port=4
  beta (rad) : Inport  Port=5
  eta_target (rad) : Inport  Port=6
  1/stick length (m^-1) : Gain  Gain=1/0.395
  Constant2 : Constant  Value=alpha0_ce
  Divide{,1..2,4} (4 alike) : Product  Inputs=*/
  Divide3 : Product  Inputs=**
  Gain : Gain  Gain=m_ce*g_ce
  Gain1 : Gain  Gain=0.5*rho_ce*s_w_ce
  Gain2 : Gain  Gain=1.75
  Gain3 : Gain  Gain=b1_ce
  Gain4 : Gain  Gain=b2_ce
  Gain5 : Gain  Gain=b3_ce
  Gain6 : Gain  Gain=0.5*rho_ce*s_e_ce*c_e_ce
  Gearing Factor (dim) : Gain  Gain=G_ce
  Square : Math  Operator=square  SaturateOnIntegerOverflow=on
  Sum{,1,3..6} (6 alike) : Sum  Inputs=|++
  Sum2 : Sum  Inputs=|+-
  Sum7 : Sum  Inputs=|+-
  downwash slope : Constant  Value=((pi*AR_w_ce*(tr_ce*r_ce)^0.25))* (1+modM_ce)
  elevator horn length (m) : Constant  Value=l_m_ce
  stick hinge moment arm length (m) : Gain  Gain=l_m_ce
  tail setting angle (rad) : Constant  Value=alpha_ts_ce
  total aircraft lift curve slope (rad^-1) : Constant  Value=dCLtot_dalpha_ce
  wing lift curve slope (rad^-1) : Gain  Gain=dCL_w_dalpha_ce
  wing setting angle (rad) : Constant  Value=alpha_ws_ce
  cessna stick force (N) : Outport
  wires:
  stick hinge moment arm length (m)/1 -> 1/stick length (m^-1)/1
  Sum/1 -> Sum7/1
  Square/1 -> Gain1/1, Divide3/2  "Vinf_t^2"
  Constant2/1 -> Sum7/2
  Gain2/1 -> Divide2/1
  Gain1/1 -> Divide/2
  total aircraft lift curve slope (rad^-1)/1 -> Divide1/2
  tail setting angle (rad)/1 -> Sum1/2
  Gain4/1 -> Sum3/2
  1/stick length (m^-1)/1 -> cessna stick force (N)/1
  Sum2/1 -> Gain3/1  "alpha_tp_eff_t (rad)"
  Gain/1 -> Divide/1
  Sum3/1 -> Sum4/1
  Divide3/1 -> Gearing Factor (dim)/1  "Mh (Nm)"
  Load Factor (dim)/1 -> Gain/1
  beta (rad)/1 -> Gain5/1
  Gain6/1 -> Divide3/1
  wing setting angle (rad)/1 -> Sum/2
  Sum1/1 -> Sum2/1  "alpha_t_t (rad), tailplane angle of attack"
  Gain3/1 -> Sum3/1
  Sum7/1 -> wing lift curve slope (rad^-1)/1
  Divide2/1 -> Sum2/2  "epsilon_t (rad)"
  wing lift curve slope (rad^-1)/1 -> Gain2/1  "CLw_t"
  Divide/1 -> Divide1/1  "CLtot (dim)"
  Gain5/1 -> Sum4/2
  Target Aircraft Flightspeed (m/s)/1 -> Square/1
  alpha0tot (rad)/1 -> Sum6/2
  Divide1/1 -> Sum6/1
  Sum6/1 -> Sum1/1, Sum/1  "alpha_fuselage_t (rad)"
  Gearing Factor (dim)/1 -> Divide4/1
  elevator horn length (m)/1 -> Divide4/2
  downwash slope/1 -> Divide2/2
  Sum4/1 -> Gain6/1  "Ch"
  Divide4/1 -> stick hinge moment arm length (m)/1  "Force in elevator linkage system (N)"
  eta (rad)/1 -> Sum5/1
  Sum5/1 -> Gain4/1
  eta_target (rad)/1 -> Sum5/2
